simulink model "simple_pid_simulink_model"  (R2021b)
settings: Solver=VariableStepAuto  StartTime=0.0  StopTime=10.0  RelTol=1e-3
settings Model: Creator=rcmas  LastModifiedBy=rcmas

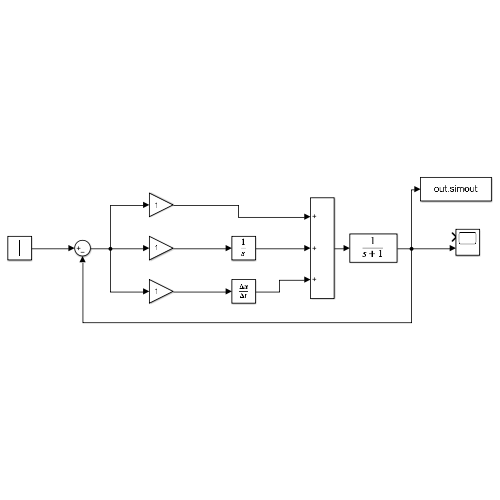
[thumbnail: Simulink's stored preview of the top-level diagram]
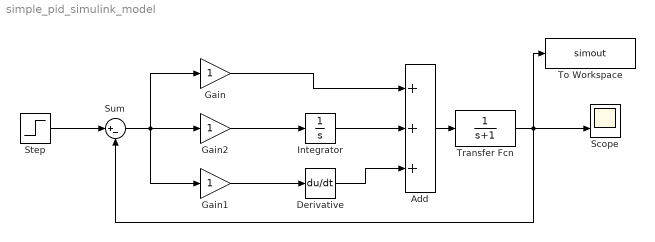
== system simple_pid_simulink_model ==
  Add : Sum  Inputs=+++
  Derivative : Derivative
  Gain : Gain
  Gain1 : Gain
  Gain2 : Gain
  Integrator : Integrator
  Scope : Scope  NumInputPorts=2
  Step : Step  Time=0  SampleTime=0
  Sum : Sum  Inputs=|+-
  To Workspace : ToWorkspace  VariableName=simout  SaveFormat=Timeseries  SampleTime=-1
      settings: StopFcn=|
      | t=out.simout.Time(:,1);
      | y=out.simout.Data(:,1);
      | plot(t,y);
  Transfer Fcn : TransferFcn  Denominator=[1 1]
  wires:
  Integrator/1 -> Add/2
  Derivative/1 -> Add/3
  Gain/1 -> Add/1
  Gain2/1 -> Integrator/1
  Gain1/1 -> Derivative/1
  Step/1 -> Sum/1
  Add/1 -> Transfer Fcn/1
  Sum/1 -> Gain1/1, Gain/1, Gain2/1
  Transfer Fcn/1 -> Scope/2, To Workspace/1, Sum/2
